simulink model "PositionComplementary"  (Simulink 6.6)
settings: Solver=ode4  StartTime=0.0  StopTime=60  FixedStep=SampleT  RelTol=1e-3
InitFcn:
  | clc
  | Taxi_Var_new
  | failures
  | insInit
  | piccolo_init
values from neighbouring files (symbols this model uses):
  A1 = 0    [Taxi_Var.m]    (also in Taxi_Var_new.m = 0.007)
  Apolar = 0.0899    [Taxi_Var.m]    (also in Taxi_Var_new.m = 0.057)
  CD0 = 0.0219    [Taxi_Var.m]    (also in Taxi_Var_new.m = 0.022)
  chord = S/span    (= 0.384036716878)    [Taxi_Var.m]    (also in Taxi_Var_new.m = 0.351341681574)
  CL0 = 0.1857    [Taxi_Var.m]    (also in Taxi_Var_new.m = 0.38)
  CLa = 4.6206    [Taxi_Var.m]    (also in Taxi_Var_new.m = 18.5)
  CLa_dot = 1.93    [Taxi_Var.m]    (also in Taxi_Var_new.m = 2.64)
  Clb = -0.0043    [Taxi_Var.m]    (also in Taxi_Var_new.m = -0.06)
  ClDa = 0.1695    [Taxi_Var.m]    (also in Taxi_Var_new.m)
  CLDe = 0.4032    [Taxi_Var.m]    (also in Taxi_Var_new.m = 0.24)
  CLDf = 0.047    [Taxi_Var.m]    (also in Taxi_Var_new.m = 0.4)
  ClDr = 0.0003    [Taxi_Var.m]    (also in Taxi_Var_new.m = 0.055)
  Clp = -0.4425    [Taxi_Var.m]    (also in Taxi_Var_new.m = -0.88)
  CLq = 8.7465    [Taxi_Var.m]    (also in Taxi_Var_new.m = 7.4)
  Clr = 0.0675    [Taxi_Var.m]    (also in Taxi_Var_new.m = 0.04)
  Cm0 = -0.0902    [Taxi_Var.m]    (also in Taxi_Var_new.m = 0.56)
  Cma = -1.3995    [Taxi_Var.m]    (also in Taxi_Var_new.m = -1.58)
  CmDe = -0.9493    [Taxi_Var.m]    (also in Taxi_Var_new.m = -41)
  CmDf = -.021    (= -0.021)    [Taxi_Var.m]    (also in Taxi_Var_new.m)
  Cmq = -10.8760    (= -10.876)    [Taxi_Var.m]    (also in Taxi_Var_new.m = -12)
  Cnb = 0.0281    [Taxi_Var.m]    (also in Taxi_Var_new.m = 0.73)
  CnDa = -0.0031    [Taxi_Var.m]    (also in Taxi_Var_new.m = -0.032)
  CnDr = -0.0882    [Taxi_Var.m]    (also in Taxi_Var_new.m = 0.19)
  Cnp = -0.0695    [Taxi_Var.m]    (also in Taxi_Var_new.m = -0.1)
  Cnr = -0.1045    [Taxi_Var.m]    (also in Taxi_Var_new.m = -0.23)
  CYb = -0.1999    [Taxi_Var.m]    (also in Taxi_Var_new.m = -0.98)
  CYDr = 0.0192    [Taxi_Var.m]    (also in Taxi_Var_new.m = 0.066)
  damax = 25*deg2rad    (= 0.436332312999)    [Taxi_Var.m]    (also in piccolo_init.m)
  damin = -25*deg2rad    (= -0.436332312999)    [Taxi_Var.m]    (also in piccolo_init.m)
  datrim = 0*deg2rad    (= 0)    [Taxi_Var.m]    (also in piccolo_init.m)
  demax = 15*deg2rad    (= 0.261799387799)    [Taxi_Var.m]    (also in piccolo_init.m)
  demin = -15*deg2rad    (= -0.261799387799)    [Taxi_Var.m]    (also in piccolo_init.m)
  detrim = -2.4137*deg2rad    (= -0.0421270121554)    [Taxi_Var.m]    (also in piccolo_init.m = -0.0523598775598)
  dfland = 30*deg2rad    (= 0.523598775598)    [Taxi_Var.m]    (also in piccolo_init.m)
  dfmax = 30*deg2rad    (= 0.523598775598)    [Taxi_Var.m]    (also in piccolo_init.m)
  dfmin = 0*deg2rad    (= 0)    [Taxi_Var.m]    (also in piccolo_init.m)
  drmax = 25*deg2rad    (= 0.436332312999)    [Taxi_Var.m]    (also in piccolo_init.m)
  drmin = -25*deg2rad    (= -0.436332312999)    [Taxi_Var.m]    (also in piccolo_init.m)
  drtrim = 0*deg2rad    (= 0)    [Taxi_Var.m]    (also in piccolo_init.m)
  dtmax = 1    [Taxi_Var.m]    (also in piccolo_init.m = 0.7)
  dtmin = 0    [Taxi_Var.m]    (also in piccolo_init.m = 0.25)
  dttrim = 0.0725    [Taxi_Var.m]    (also in piccolo_init.m = 0.35)
  Euler_0 = [0; 0; 45]'*pi/180    [Taxi_Var.m]    (also in Taxi_Var_new.m = [0 0 45]'*pi/180)
  IdxCmdOrbitRadius = 17    [piccolo_init.m]
  IdxCmdOrbitSense = 18    [piccolo_init.m]
  IdxCmdWp1Alt = 13    [piccolo_init.m]
  IdxCmdWp1Lat = 11    [piccolo_init.m]
  IdxCmdWp1Lon = 12    [piccolo_init.m]
  IdxCmdWp2Alt = 16    [piccolo_init.m]
  IdxCmdWp2Lat = 14    [piccolo_init.m]
  IdxCmdWp2Lon = 15    [piccolo_init.m]
  IdxEstimReserved1 = 4    [piccolo_init.m]
  IdxEstimWEast = 3    [piccolo_init.m]
  IdxEstimWNorth = 2    [piccolo_init.m]
  IdxGainsAltD = 10    [piccolo_init.m]
  IdxGainsAltI = 9    [piccolo_init.m]
  IdxGainsAltP = 8    [piccolo_init.m]
  IdxGainsPdynD = 4    [piccolo_init.m]
  IdxGainsPdynI = 3    [piccolo_init.m]
  IdxGainsPdynP = 2    [piccolo_init.m]
  IdxGainsPitchD = 7    [piccolo_init.m]
  IdxGainsPitchI = 6    [piccolo_init.m]
  IdxGainsPitchP = 5    [piccolo_init.m]
  IdxGainsRollD = 17    [piccolo_init.m]
  IdxGainsRollI = 16    [piccolo_init.m]
  IdxGainsRollP = 15    [piccolo_init.m]
  IdxGainsSlopeElevatorD = 25    [piccolo_init.m]
  IdxGainsSlopeElevatorP = 26    [piccolo_init.m]
  IdxGainsTrackConv = 24    [piccolo_init.m]
  IdxGainsTrackD = 23    [piccolo_init.m]
  IdxGainsTrackI = 22    [piccolo_init.m]
  IdxGainsTrackP = 21    [piccolo_init.m]
  IdxGainsTurnD = 14    [piccolo_init.m]
  IdxGainsTurnI = 13    [piccolo_init.m]
  IdxGainsTurnP = 12    [piccolo_init.m]
  IdxGainsYawD = 20    [piccolo_init.m]
  IdxGainsYawI = 19    [piccolo_init.m]
  IdxGainsYawP = 18    [piccolo_init.m]
  IdxLimitsAileronMax = 11    [piccolo_init.m]
  IdxLimitsAileronMin = 10    [piccolo_init.m]
  IdxLimitsBankMax = 9    [piccolo_init.m]
  IdxLimitsBankMin = 8    [piccolo_init.m]
  IdxLimitsElevatorMax = 13    [piccolo_init.m]
  IdxLimitsElevatorMin = 12    [piccolo_init.m]
  IdxLimitsFlapMax = 19    [piccolo_init.m]
  IdxLimitsFlapMin = 18    [piccolo_init.m]
  IdxLimitsPdynMax = 3    [piccolo_init.m]
  IdxLimitsPdynMin = 2    [piccolo_init.m]
  IdxLimitsRudderMax = 15    [piccolo_init.m]
  IdxLimitsRudderMin = 14    [piccolo_init.m]
  IdxLimitsThrottleMax = 17    [piccolo_init.m]
  IdxLimitsThrottleMin = 16    [piccolo_init.m]
  IdxSensorsAlt = 5    [piccolo_init.m]
  IdxSensorsLat = 3    [piccolo_init.m]
  IdxSensorsLon = 4    [piccolo_init.m]
  IdxSensorsVDown = 8    [piccolo_init.m]
  IdxSensorsVEast = 7    [piccolo_init.m]
  IdxSensorsVNorth = 6    [piccolo_init.m]
  IdxStatesGlobal = 2    [piccolo_init.m]
  IdxStatesManual = 16    [piccolo_init.m]
  IdxStatesMode = 15    [piccolo_init.m]
  ISA_g = 9.815    [Taxi_Var.m]    (also in Taxi_Var_new.m)
  ISA_hmax = 2000    [Taxi_Var.m]    (also in Taxi_Var_new.m)
  ISA_lapse = .0065    (= 0.0065)    [Taxi_Var.m]    (also in Taxi_Var_new.m)
  ISA_P0 = 101325    [Taxi_Var.m]    (also in Taxi_Var_new.m)
  ISA_R = 287    [Taxi_Var.m]    (also in Taxi_Var_new.m)
  ISA_rho0 = 1.225    [Taxi_Var.m]    (also in Taxi_Var_new.m)
  ISA_T0 = 289    [Taxi_Var.m]    (also in Taxi_Var_new.m)
  Ixx = 3.689084    [Taxi_Var.m]    (also in Taxi_Var_new.m = 3.8)
  Iyy = 7.43789    [Taxi_Var.m]    (also in Taxi_Var_new.m = 9.58)
  Izz = 10.22202    [Taxi_Var.m]    (also in Taxi_Var_new.m = 9.68)
  mass = 22.5    [Taxi_Var.m]    (also in Taxi_Var_new.m = 8.16466266)
  MinThK = 0.075    [Taxi_Var.m]    (also in Taxi_Var_new.m = 0.077)
  Pos_0 = [0; 0; 1000]'    [Taxi_Var.m]    (also in Taxi_Var_new.m = [0 0 500]')
  PQR_0 = [0; 0; 0]'    [Taxi_Var.m]    (also in Taxi_Var_new.m = [ 0 0 0]'*pi/180)
  SampleT = 0.005    [failures.m]
  span = 2.3368    [Taxi_Var.m]    (also in Taxi_Var_new.m = 2.795)
  TFact = 0.4    [Taxi_Var.m]    (also in Taxi_Var_new.m)
  ThK = 2.18    [Taxi_Var.m]    (also in Taxi_Var_new.m = 2.17)
  tsamp = APtsamp    (= 0.05)    [piccolo_init.m]
  ... (+1 more)
undefined symbols (not defined in the file or in its folder): clock, Earth, gaind, polesd, WGS84, zerosd
libraries: piccolo_library x60, simulink x45, aerolibconvert2 x13, dspsigops x5, aerolibasang x5, aerolibatmos2 x2, aerolibtransform2 x2, aerolibnav x2, aerolibutil x1, dspmtrx3 x1
(part 4 of 5)

== system PositionComplementary/Plant Model/Plant/6-DOF EOM/[V1,2,3,W1,2,3] ==
  note: V*dot =Inv(A){[F ; M] - SigmaAV*}
  "[F ; M]" : Inport
  Euler : Inport  Port=2
  V* : Inport  Port=3  PortDimensions=6
  A = [M ; J] : Subsystem
  Acc_meas : Product  Inputs=/*  Multiplication=Matrix(*)  SaturateOnIntegerOverflow=on  InputSameDT=on
  Demux : Demux  Outputs=[3;3]
  Get Grav Force in Body : Subsystem
  Gravitational Acc : Constant  Value=[0 0 -ISA_g]  VectorParams1D=off
  Reshape1 : Reshape
  Reshape2 : Reshape
  Scope : Scope
      settings: YMin=-90  YMax=10  SaveName=ScopeData34
  Selector3 : Selector  IndexOptions=Index vector (dialog)  Indices=1:3  OutputSizes=1  InputPortWidth=6
  Sigma : Subsystem
  Sigma*A : Product  Multiplication=Matrix(*)  SaturateOnIntegerOverflow=on  InputSameDT=on
  Sigma*A*V* : Product  Multiplication=Matrix(*)  SaturateOnIntegerOverflow=on  InputSameDT=on
  Sum1 : Sum  Inputs=+-|  SaturateOnIntegerOverflow=on  InputSameDT=on
  Sum2 : Sum  Inputs=++|  SaturateOnIntegerOverflow=on  InputSameDT=on
  Terminator1 : Terminator
  "V*dot " : Product  Inputs=/*  Multiplication=Matrix(*)  SaturateOnIntegerOverflow=on  InputSameDT=on
  "Acc_meas " : Outport
  V*dot : Outport  Port=2
  wires:
  Sum2/1 -> Reshape2/1
  Get Grav Force in Body/1(Grav Force (Body)) -> Reshape1/1
  Selector3/1 -> Sum2/2
  Euler/1 -> Get Grav Force in Body/1(Euler)
  Gravitational Acc/1 -> Get Grav Force in Body/2(Grav Force)
  Acc_meas/1 -> Selector3/1
  Sigma*A/1 -> Sigma*A*V*/1
  "V*dot "/1 -> V*dot/1
  V*/1 -> Demux/1, Sigma*A*V*/2
  Demux/2 -> Sigma/1(pqr)
  Sigma*A*V*/1 -> Sum1/2
  "[F ; M]"/1 -> Acc_meas/2, Sum1/1
  Sigma/1(Sigma) -> Sigma*A/1
  Demux/1 -> Terminator1/1
  A = [M ; J]/1(A Matrix) -> Acc_meas/1, "V*dot "/1, Sigma*A/2
  Sum1/1 -> "V*dot "/2
  Reshape1/1 -> Sum2/1
  Reshape2/1 -> "Acc_meas "/1, Scope/1

== system PositionComplementary/Plant Model/Plant/Engine Model/Get To1 ==
  dt : Inport
  Divide : Product  Inputs=3  OutScaling=2^-10
  Math Function : Math  Operator=pow  SaturateOnIntegerOverflow=on
  Math Function1 : Math  Operator=pow  SaturateOnIntegerOverflow=on
  MaxRPM : Gain  Gain=7200  SaturateOnIntegerOverflow=on
  Min RPM : Constant  Value=2000
  Min Th K : Constant  Value=MinThK
  Prop Diameter (in) : Constant  Value=17
  Prop Diameter (in)1 : Constant  Value=2
  Prop Diameter (in)2 : Constant  Value=4
  Saturation : Saturate  UpperLimit=1.0  LowerLimit=0.2
  Sum : Sum  Inputs=|++
  Sum1 : Sum  Inputs=|++
  TFact : simulink/Math Operations/Slider Gain  SystemSampleTime=-1  low=0  gain=0.2  high=1
  "TFact " : Gain  Gain=TFact  SaturateOnIntegerOverflow=on
  Th K : Gain  Gain=ThK  SaturateOnIntegerOverflow=on
  To Constant : Constant  Value=2.83e-12
  RPM : Outport
  To : Outport  Port=2
  wires:
  Saturation/1 -> Th K/1
  Prop Diameter (in)1/1 -> Math Function/2
  Prop Diameter (in)2/1 -> Math Function1/2
  Prop Diameter (in)/1 -> Math Function1/1
  Math Function/1 -> Divide/1
  Math Function1/1 -> Divide/2
  To Constant/1 -> Divide/3
  Divide/1 -> TFact/1
  TFact/1 -> To/1
  Sum/1 -> Math Function/1, RPM/1
  Min RPM/1 -> Sum/2
  MaxRPM/1 -> Sum/1
  Th K/1 -> Sum1/1
  dt/1 -> Saturation/1
  Sum1/1 -> MaxRPM/1
  Min Th K/1 -> Sum1/2

== system PositionComplementary/Plant Model/Plant/Forces and Moments/Alpha/Beta ==
  "Vx, Vy, Vz (Body)" : Inport
  Rho : Inport  Port=2
  Constant : Constant  Value=0.5  VectorParams1D=off
  Math Function : Math  Operator=sqrt  SaturateOnIntegerOverflow=on
  Product : Product  Inputs=3  SaturateOnIntegerOverflow=on
  Product1 : Product  Inputs=3  SaturateOnIntegerOverflow=on
  R2D1 : Gain  Gain=180/pi  SaturateOnIntegerOverflow=on
  R2D2 : Gain  Gain=180/pi  SaturateOnIntegerOverflow=on
  V^2 : Fcn  Expr=(u(1)^2+u(2)^2+u(3)^2)
  "[-15; 15 ]" : Saturate  UpperLimit=15  LowerLimit=-15
  "[-15;15]" : Saturate  UpperLimit=15  LowerLimit=-15
  aoa : Trigonometry  Operator=asin
  beta : Trigonometry  Operator=atan
  sin(aoa) : Fcn  Expr=u(3)/sqrt(u(1)^2+u(3)^2)
  span : Constant  Value=span  VectorParams1D=off
  span1 : Constant  Value=chord  VectorParams1D=off
  tan(beta) : Fcn  Expr=u(2)/sqrt(u(1)^2+u(3)^2)
  "alpha, deg" : Outport
  "beta, deg" : Outport  Port=2
  qS : Outport  Port=3
  Speed : Outport  Port=4
  q : Outport  Port=5
  wires:
  Product/1 -> q/1, Product1/1
  Product1/1 -> qS/1
  span1/1 -> Product1/3
  span/1 -> Product1/2
  "Vx, Vy, Vz (Body)"/1 -> sin(aoa)/1, V^2/1, tan(beta)/1
  tan(beta)/1 -> beta/1
  beta/1 -> R2D1/1
  V^2/1 -> Product/1, Math Function/1
  Rho/1 -> Product/2
  Constant/1 -> Product/3
  R2D1/1 -> "[-15; 15 ]"/1  "beta"
  aoa/1 -> R2D2/1
  R2D2/1 -> "[-15;15]"/1  "aoa"
  sin(aoa)/1 -> aoa/1
  Math Function/1 -> Speed/1
  "[-15;15]"/1 -> "alpha, deg"/1
  "[-15; 15 ]"/1 -> "beta, deg"/1

== system PositionComplementary/Plant Model/Plant/Forces and Moments/Body Frame F & M ==
  "Alpha, deg" : Inport
  "Beta, deg" : Inport  Port=2
  qs : Inport  Port=3
  Airspeed : Inport  Port=4
  "de, deg" : Inport  Port=5
  "da, deg" : Inport  Port=6
  "dr, deg" : Inport  Port=7
  "df, deg" : Inport  Port=8
  p,q,r : Inport  Port=9
  Bus Creator : BusCreator  Inputs=2
  Transfer to body frame : Subsystem
  Wind frame F& M : Subsystem
  F_b : Outport
  M_b : Outport  Port=2
  wires:
  "Alpha, deg"/1 -> Wind frame F& M/1("alpha, deg"), Bus Creator/1
  "Beta, deg"/1 -> Wind frame F& M/2("beta, deg"), Bus Creator/2
  "dr, deg"/1 -> Wind frame F& M/5("dr, deg")
  "da, deg"/1 -> Wind frame F& M/4("da, deg")
  "de, deg"/1 -> Wind frame F& M/3("de, deg")
  Wind frame F& M/1(F&M wind frame) -> Transfer to body frame/1(Wind frame  F&M)
  Bus Creator/1 -> Transfer to body frame/2("aoa/beta, deg")  "aoa/beta, deg"
  Transfer to body frame/1(F_b) -> F_b/1
  Transfer to body frame/2(M_b) -> M_b/1
  "df, deg"/1 -> Wind frame F& M/6("df, deg")
  qs/1 -> Wind frame F& M/7(qS)
  p,q,r/1 -> Wind frame F& M/8(p,q,r)
  Airspeed/1 -> Wind frame F& M/9(Airpseed)

== system PositionComplementary/Plant Model/Plant/Forces and Moments/Get Grav Force in Body ==
  Euler : Inport
  Grav Force : Inport  Port=2
  Math Function : Math  Operator=transpose  SaturateOnIntegerOverflow=on
  Product1 : Product  Multiplication=Matrix(*)  SaturateOnIntegerOverflow=on  InputSameDT=on
  Rb2u : Subsystem
  Reshape : Reshape  OutputDimensionality=Column vector (2-D)
  Grav Force (Body) : Outport
  wires:
  Rb2u/1(DCM) -> Math Function/1
  Euler/1 -> Rb2u/1(phi theta psi)
  Product1/1 -> Grav Force (Body)/1
  Math Function/1 -> Product1/1
  Grav Force/1 -> Reshape/1
  Reshape/1 -> Product1/2

== system PositionComplementary/Plant Model/Plant/Forces and Moments/NED(u)2b ==
  V w : Inport
  Euler : Inport  Port=2
  RB2LTP : Subsystem
  RL2B * Vw : Product  Multiplication=Matrix(*)  SaturateOnIntegerOverflow=on  InputSameDT=on
  RLTP2B : Math  Operator=transpose  SaturateOnIntegerOverflow=on
  Reshape1 : Reshape  OutputDimensionality=Row vector (2-D)
  Vb Corr : Outport
  wires:
  RL2B * Vw/1 -> Reshape1/1
  Euler/1 -> RB2LTP/1(Euler)
  RB2LTP/1(RB2L) -> RLTP2B/1
  RLTP2B/1 -> RL2B * Vw/1
  V w/1 -> RL2B * Vw/2
  Reshape1/1 -> Vb Corr/1

== system PositionComplementary/Signal Cond/Accel Convert/3vector LPF/Low Pass1 ==
  In1 : Inport
  Discrete Zero-Pole : DiscreteZeroPole  Zeros=zerosd  Poles=polesd  Gain=gaind  SampleTime=SampleTime
  Out1 : Outport
  wires:
  In1/1 -> Discrete Zero-Pole/1
  Discrete Zero-Pole/1 -> Out1/1

== system PositionComplementary/Signal Cond/Accel Convert/3vector LPF/Low Pass2 ==
  In1 : Inport
  Discrete Zero-Pole : DiscreteZeroPole  Zeros=zerosd  Poles=polesd  Gain=gaind  SampleTime=SampleTime
  Out1 : Outport
  wires:
  Discrete Zero-Pole/1 -> Out1/1
  In1/1 -> Discrete Zero-Pole/1

== system PositionComplementary/Signal Cond/Accel Convert/3vector LPF/Low Pass3 ==
  In1 : Inport
  Discrete Zero-Pole : DiscreteZeroPole  Zeros=zerosd  Poles=polesd  Gain=gaind  SampleTime=SampleTime
  Out1 : Outport
  wires:
  In1/1 -> Discrete Zero-Pole/1
  Discrete Zero-Pole/1 -> Out1/1

== system PositionComplementary/Signal Cond/Gyro Convert/3vector LPF/Low Pass1 ==
  In1 : Inport
  Discrete Zero-Pole : DiscreteZeroPole  Zeros=zerosd  Poles=polesd  Gain=gaind  SampleTime=SampleTime
  Out1 : Outport
  wires:
  In1/1 -> Discrete Zero-Pole/1
  Discrete Zero-Pole/1 -> Out1/1

== system PositionComplementary/Signal Cond/Gyro Convert/3vector LPF/Low Pass2 ==
  In1 : Inport
  Discrete Zero-Pole : DiscreteZeroPole  Zeros=zerosd  Poles=polesd  Gain=gaind  SampleTime=SampleTime
  Out1 : Outport
  wires:
  Discrete Zero-Pole/1 -> Out1/1
  In1/1 -> Discrete Zero-Pole/1

== system PositionComplementary/Signal Cond/Gyro Convert/3vector LPF/Low Pass3 ==
  In1 : Inport
  Discrete Zero-Pole : DiscreteZeroPole  Zeros=zerosd  Poles=polesd  Gain=gaind  SampleTime=SampleTime
  Out1 : Outport
  wires:
  In1/1 -> Discrete Zero-Pole/1
  Discrete Zero-Pole/1 -> Out1/1

== system PositionComplementary/Subsystem3/Autopilot/Altitude Control Vector Inputs/Alt switch ==
  note: Select whether the individual components of the altitude, airspeed and turn rate loops are enabled or
      | disabled.  This is done based on the specific loop enable state, the global state, and the mode of the autopilot.
      |
      | Note the use of the multiport  switch.  This switch is one based, and will truncate floating point
      | numbers.  Hence we add by 1.1 to guarantee we don't get the wrong state based on rounding
      | error.
  Globals : Inport
  Loop : Inport  Port=2
  Climbout : Constant
  Convert to 1 based : Constant  Value=1.1
  Default : Constant
  Demux : Demux  Outputs=3
  Display4 : Display
  Final Approach : Constant
  Flying : Constant
  Global and Loop on/off : Product  SaturateOnIntegerOverflow=on
  Land pattern : Constant
  Loop on or off : Switch  Threshold=0.5  SaturateOnIntegerOverflow=on
  Mux : Mux  Inputs=3
  Mux1 : Mux  Inputs=3
  PID switch : MultiPortSwitch  Inputs=8  SaturateOnIntegerOverflow=on  InputSameDT=on
  Pre launch : Constant  Value=0
  Sum : Sum  Inputs=++|  SaturateOnIntegerOverflow=on  InputSameDT=on
  Terminator : Terminator
  Touchdown : Constant
  Transition : Constant  Value=0
  Zero : Constant  Value=0
  TriOut : Outport  OutDataType=fixdt(1,16,0)  OutScaling=[]
  wires:
  Sum/1 -> PID switch/1
  Default/1 -> PID switch/9
  Touchdown/1 -> PID switch/8
  Final Approach/1 -> PID switch/7
  Land pattern/1 -> PID switch/6
  Flying/1 -> PID switch/5
  Transition/1 -> PID switch/3
  Climbout/1 -> PID switch/4
  Pre launch/1 -> PID switch/2
  Demux/3 -> Terminator/1
  Mux1/1 -> Loop on or off/1
  PID switch/1 -> Mux1/3, Mux1/2, Mux1/1
  Convert to 1 based/1 -> Sum/1
  Demux/2 -> Sum/2
  Global and Loop on/off/1 -> Loop on or off/2
  Loop/1 -> Global and Loop on/off/2
  Demux/1 -> Global and Loop on/off/1
  Globals/1 -> Demux/1, Display4/1
  Zero/1 -> Mux/3, Mux/2, Mux/1
  Mux/1 -> Loop on or off/3
  Loop on or off/1 -> TriOut/1

== system PositionComplementary/Subsystem3/Autopilot/Altitude Control Vector Inputs/Integral Gain  Scheduling ==
  note: 3. Then the IntegralGain2 = IntegralGain * GainScheduleFactor
  note: 2. We compute GainScheduleFactor = exp(-error^2 / (2*sigma^2))
  note: 1. We compute sigma = ScalingParam * ActuatorRange/2 / Kp
  note: Integral gain scheduling based on a Gaussian distribution, as a function of the error, actuator range, and proportional gain.
  err : Inport
  Gains : Inport  Port=2
  Limits : Inport  Port=3
  Demux : Demux  Outputs=2
  Demux1 : Demux  Outputs=3
  Gain : Gain  Gain=0.5  SaturateOnIntegerOverflow=on
  Gain1 : Gain  Gain=2  SaturateOnIntegerOverflow=on
  Gain2 : Gain  Gain=-1  SaturateOnIntegerOverflow=on
  Math Function : Math  Operator=square  OutDataType=fixdt(1,16,0)  OutScaling=[]  SaturateOnIntegerOverflow=on
  Math Function1 : Math  Operator=square  OutDataType=fixdt(1,16,0)  OutScaling=[]  SaturateOnIntegerOverflow=on
  Math Function2 : Math  OutDataType=fixdt(1,16,0)  OutScaling=[]  SaturateOnIntegerOverflow=on
  Mux1 : Mux  Inputs=3
  Product : Product  Inputs=/**  SaturateOnIntegerOverflow=on
  Product1 : Product  Inputs=*/  SaturateOnIntegerOverflow=on
  Product2 : Product  SaturateOnIntegerOverflow=on
  Scaling param : Constant  Value=0.5
  Sum : Sum  Inputs=+-  SaturateOnIntegerOverflow=on
  Zero Protect : piccolo_library/Math/Zero Protect  SystemSampleTime=-1  p=1  tol=1e-6
  Gains2 : Outport  OutDataType=fixdt(1,16,0)  OutScaling=[]
  wires:
  Zero Protect/1 -> Product/1
  Demux1/1 -> Mux1/1, Zero Protect/1
  Demux1/3 -> Mux1/3
  Product2/1 -> Mux1/2
  Mux1/1 -> Gains2/1
  Demux1/2 -> Product2/2
  Gains/1 -> Demux1/1
  Math Function2/1 -> Product2/1
  Product1/1 -> Math Function2/1
  Gain1/1 -> Product1/2
  Gain2/1 -> Product1/1
  Math Function1/1 -> Gain2/1
  err/1 -> Math Function1/1
  Math Function/1 -> Gain1/1
  Product/1 -> Math Function/1
  Scaling param/1 -> Product/3
  Gain/1 -> Product/2
  Sum/1 -> Gain/1
  Demux/2 -> Sum/2
  Demux/1 -> Sum/1
  Limits/1 -> Demux/1

== system PositionComplementary/Subsystem3/Autopilot/Altitude Control Vector Inputs/Min alt ==
  note: Determin the min altitude to use. Either -10000 or the passed in value, depending on if Auto land is enabled
  Globals : Inport
  MinAlt : Inport  Port=2
  -10000 : Constant  Value=-10000
  Climbout : Constant  Value=0
  Convert to 1 based : Constant  Value=1.1
  Default : Constant  Value=0
  Demux : Demux  Outputs=3
  Final Approach : Constant
  Flying : Constant  Value=0
  Land pattern : Constant
  Loop on or off : Switch  Threshold=0.5  SaturateOnIntegerOverflow=on
  Min alt on/off : MultiPortSwitch  Inputs=8  SaturateOnIntegerOverflow=on  InputSameDT=on
  Pre launch : Constant  Value=0
  Sum : Sum  Inputs=++|  SaturateOnIntegerOverflow=on  InputSameDT=on
  Terminator : Terminator
  Terminator1 : Terminator
  Touchdown : Constant
  Transition : Constant  Value=0
  MinAltOut : Outport  OutDataType=fixdt(1,16,0)  OutScaling=[]
  wires:
  Sum/1 -> Min alt on/off/1
  Default/1 -> Min alt on/off/9
  Touchdown/1 -> Min alt on/off/8
  Final Approach/1 -> Min alt on/off/7
  Land pattern/1 -> Min alt on/off/6
  Flying/1 -> Min alt on/off/5
  Transition/1 -> Min alt on/off/3
  Climbout/1 -> Min alt on/off/4
  Pre launch/1 -> Min alt on/off/2
  -10000/1 -> Loop on or off/1
  Min alt on/off/1 -> Loop on or off/2
  Loop on or off/1 -> MinAltOut/1
  Globals/1 -> Demux/1
  Demux/1 -> Terminator1/1
  MinAlt/1 -> Loop on or off/3
  Demux/2 -> Sum/2
  Convert to 1 based/1 -> Sum/1
  Demux/3 -> Terminator/1

== system PositionComplementary/Subsystem3/Autopilot/Altitude Control Vector Inputs/PID Controller ==
  note: Standard PID feedback controller with integrator saturation. There are three gains, and three states, one for each term
  Input : Inport
  Cmd : Inport  Port=2
  State : Inport  Port=3
  Gains : Inport  Port=4
  Limits : Inport  Port=5
  IniCond : Inport  Port=6
  Demux : Demux  Outputs=3
  Demux1 : Demux  Outputs=3
  Derivative Gain : Product  Inputs=3  SaturateOnIntegerOverflow=on  InputSameDT=on
  Extended Integrator : Subsystem  AncestorBlock=piccolo_library/Integrators/Extended Integrator  mask(Extended Integrator){T=tsamp}
      mask prompts: T "Sample time:"
      mask help:
      | Trapezoidal integration with integrator reset and anti-windup logic
      | The block computes the integral.  The integrator gets the IC value
      | whenever the enable line is down.  Anytime the enable line is
      | down the output is the IC value.  If the gain goes to zero then the
      | integrator value is reset.
  Proportional Gain : Product  Inputs=3  SaturateOnIntegerOverflow=on  InputSameDT=on
  Scope1 : Scope  NumInputPorts=3
      settings: YMin=0.045~0.038~-1  YMax=0.051~0.058~1  SaveName=ScopeData32
  Scope2 : Scope  NumInputPorts=3
      settings: YMin=0.045~0.038~-1  YMax=0.051~0.058~1  SaveName=ScopeData20
  Sum : Sum  Inputs=|+-  SaturateOnIntegerOverflow=on
  Sum3 : Sum  Inputs=+++  SaturateOnIntegerOverflow=on  InputSameDT=on
  dx/dt with TD : piccolo_library/Derivatives/dx//dt with TD  SystemSampleTime=-1  tsamp=tsamp  tdelay=tdelay
  Output : Outport  OutDataType=fixdt(1,16,0)  OutScaling=[]
  wires:
  Sum3/1 -> Output/1
  Demux1/3 -> Derivative Gain/3
  Demux1/2 -> Extended Integrator/3(Enable)
  Demux1/1 -> Proportional Gain/3
  State/1 -> Demux1/1
  IniCond/1 -> Extended Integrator/2(IniCond)
  Limits/1 -> Extended Integrator/5(Limits)
  Demux/2 -> Extended Integrator/4(Gain)
  Extended Integrator/1(Out) -> Sum3/2, Scope2/2
  Derivative Gain/1 -> Sum3/3, Scope2/3
  Proportional Gain/1 -> Sum3/1, Scope2/1
  Demux/3 -> Derivative Gain/2
  Demux/1 -> Proportional Gain/2
  Gains/1 -> Demux/1
  dx/dt with TD/1 -> Derivative Gain/1
  Sum/1 -> Extended Integrator/1(Input), dx/dt with TD/1, Proportional Gain/1
  Cmd/1 -> Sum/2, Scope1/1, Scope1/2
  Input/1 -> Sum/1

== system PositionComplementary/Subsystem3/Autopilot/Altitude Control Vector Inputs/Total Energy1 ==
  TAS : Inport
  Alt : Inport  Port=2
  TASCmd : Inport  Port=3
  AltCmd : Inport  Port=4
  State : Inport  Port=5
  1/2 : Constant  Value=0.5
  Kinetic : Product  Inputs=***  SaturateOnIntegerOverflow=on  InputSameDT=on
  Kinetic1 : Product  Inputs=*/  SaturateOnIntegerOverflow=on  InputSameDT=on
  Kinetic2 : Product  Inputs=***  SaturateOnIntegerOverflow=on  InputSameDT=on
  Sum1 : Sum  SaturateOnIntegerOverflow=on  InputSameDT=on
  Sum2 : Sum  SaturateOnIntegerOverflow=on  InputSameDT=on
  Switch : Switch  Threshold=0.5  SaturateOnIntegerOverflow=on
  Switch1 : Switch  Threshold=0.5  SaturateOnIntegerOverflow=on
  Zero : Constant  Value=0.0
  g1 : Constant  Value=9.806
  Energy : Outport  OutDataType=fixdt(1,16,0)  OutScaling=[]
  Cmd : Outport  Port=2  OutDataType=fixdt(1,16,0)  OutScaling=[]
  wires:
  TASCmd/1 -> Kinetic2/3, Kinetic2/2
  Sum1/1 -> Cmd/1
  AltCmd/1 -> Sum1/2
  Switch1/1 -> Sum1/1
  Kinetic2/1 -> Switch1/1
  Sum2/1 -> Energy/1
  Alt/1 -> Sum2/1
  Switch/1 -> Sum2/2
  Kinetic1/1 -> Kinetic2/1, Kinetic/3
  1/2/1 -> Kinetic1/1
  g1/1 -> Kinetic1/2
  Kinetic/1 -> Switch/1
  State/1 -> Switch/2, Switch1/2
  Zero/1 -> Switch/3, Switch1/3
  TAS/1 -> Kinetic/1, Kinetic/2

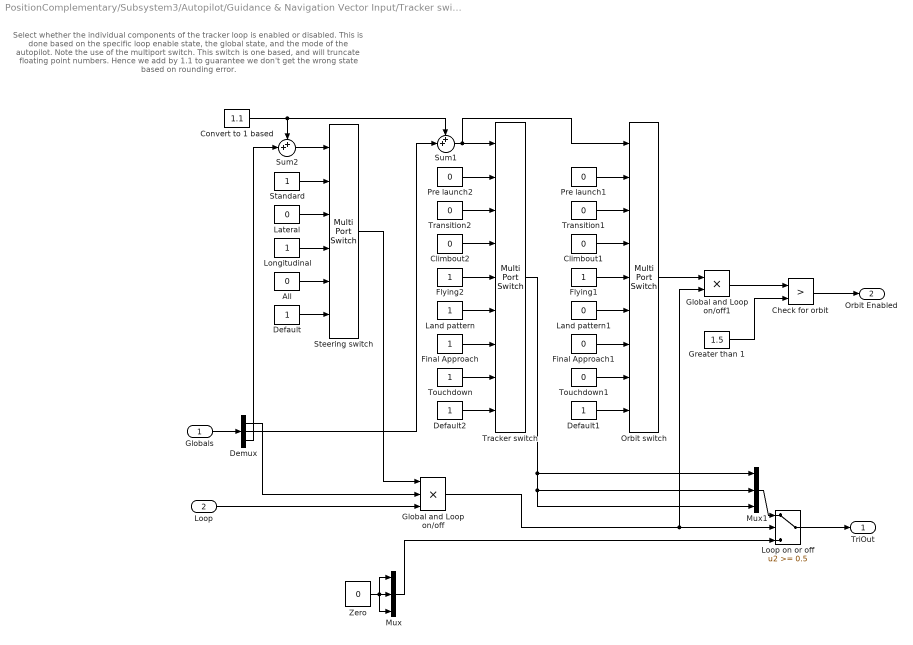
== system PositionComplementary/Subsystem3/Autopilot/Guidance & Navigation Vector Input/Tracker switch ==
  note: Select whether the individual components of the tracker loop is enabled or
      | disabled.  This is done based on the specific loop enable state, the global state, and the mode of the autopilot.
      |
      | Note the use of the multiport  switch.  This switch is one based, and will truncate floating point
      | numbers.  Hence we add by 1.1 to guarantee we don't get the wrong state based on rounding
      | error.
  Globals : Inport
  Loop : Inport  Port=2
  All : Constant  Value=0
  Check for orbit : RelationalOperator  Operator=>
  Climbout1 : Constant  Value=0
  Climbout2 : Constant  Value=0
  Convert to 1 based : Constant  Value=1.1
  Default : Constant
  Default1 : Constant
  Default2 : Constant
  Demux : Demux  Outputs=3
  Final Approach : Constant
  Final Approach1 : Constant  Value=0
  Flying1 : Constant
  Flying2 : Constant
  Global and Loop on/off : Product  Inputs=3  SaturateOnIntegerOverflow=on
  Global and Loop on/off1 : Product  SaturateOnIntegerOverflow=on
  Greater than 1 : Constant  Value=1.5
  Land pattern : Constant
  Land pattern1 : Constant  Value=0
  Lateral : Constant  Value=0
  Longitudinal : Constant
  Loop on or off : Switch  Threshold=0.5  SaturateOnIntegerOverflow=on
  Mux : Mux  Inputs=3
  Mux1 : Mux  Inputs=3
  Orbit switch : MultiPortSwitch  Inputs=8  SaturateOnIntegerOverflow=on  InputSameDT=on
  Pre launch1 : Constant  Value=0
  Pre launch2 : Constant  Value=0
  Standard : Constant
  Steering switch : MultiPortSwitch  Inputs=5  SaturateOnIntegerOverflow=on  InputSameDT=on
  Sum1 : Sum  Inputs=++|  SaturateOnIntegerOverflow=on  InputSameDT=on
  Sum2 : Sum  Inputs=++|  SaturateOnIntegerOverflow=on  InputSameDT=on
  Touchdown : Constant
  Touchdown1 : Constant  Value=0
  Tracker switch : MultiPortSwitch  Inputs=8  SaturateOnIntegerOverflow=on  InputSameDT=on
  Transition1 : Constant  Value=0
  Transition2 : Constant  Value=0
  Zero : Constant  Value=0
  TriOut : Outport  OutDataType=fixdt(1,16,0)  OutScaling=[]
  Orbit Enabled : Outport  Port=2  OutDataType=fixdt(1,16,0)  OutScaling=[]
  wires:
  Steering switch/1 -> Global and Loop on/off/1
  Demux/1 -> Global and Loop on/off/2
  Loop/1 -> Global and Loop on/off/3
  Sum2/1 -> Steering switch/1
  Default/1 -> Steering switch/6
  All/1 -> Steering switch/5
  Lateral/1 -> Steering switch/3
  Longitudinal/1 -> Steering switch/4
  Standard/1 -> Steering switch/2
  Convert to 1 based/1 -> Sum2/1, Sum1/1
  Default1/1 -> Orbit switch/9
  Touchdown1/1 -> Orbit switch/8
  Final Approach1/1 -> Orbit switch/7
  Land pattern1/1 -> Orbit switch/6
  Flying1/1 -> Orbit switch/5
  Transition1/1 -> Orbit switch/3
  Climbout1/1 -> Orbit switch/4
  Pre launch1/1 -> Orbit switch/2
  Sum1/1 -> Orbit switch/1, Tracker switch/1
  Default2/1 -> Tracker switch/9
  Touchdown/1 -> Tracker switch/8
  Final Approach/1 -> Tracker switch/7
  Land pattern/1 -> Tracker switch/6
  Flying2/1 -> Tracker switch/5
  Transition2/1 -> Tracker switch/3
  Climbout2/1 -> Tracker switch/4
  Pre launch2/1 -> Tracker switch/2
  Mux1/1 -> Loop on or off/1
  Tracker switch/1 -> Mux1/2, Mux1/3, Mux1/1
  Zero/1 -> Mux/3, Mux/2, Mux/1
  Mux/1 -> Loop on or off/3
  Check for orbit/1 -> Orbit Enabled/1
  Greater than 1/1 -> Check for orbit/2
  Orbit switch/1 -> Global and Loop on/off1/1
  Global and Loop on/off1/1 -> Check for orbit/1
  Demux/3 -> Sum2/2
  Demux/2 -> Sum1/2
  Global and Loop on/off/1 -> Global and Loop on/off1/2, Loop on or off/2
  Globals/1 -> Demux/1
  Loop on or off/1 -> TriOut/1

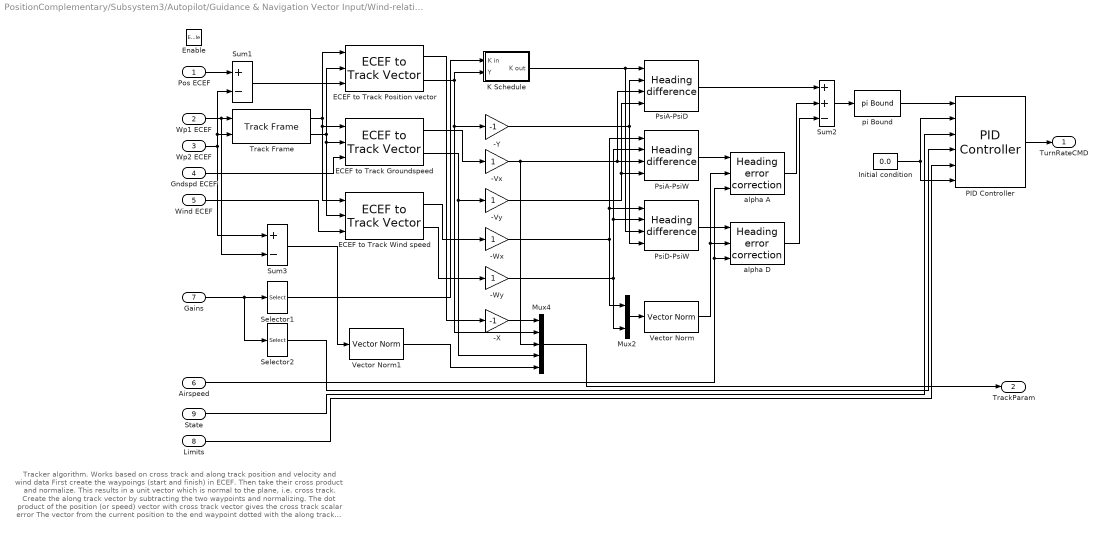
== system PositionComplementary/Subsystem3/Autopilot/Guidance & Navigation Vector Input/Wind-relative Tracker ==
  note: Tracker algorithm.  Works based on cross track and along track position and velocity and wind data
      |
      | First create the waypoings (start and finish) in ECEF.  Then take their cross product and normalize.  This results in a unit vector which is normal to the plane, i.e. cross track.
      | Create the along track vector by subtracting the two waypoints and normalizing.
      | The dot product of the position (or speed) vector with cross track vector gives the cross track scalar error
      | The vector from the current position to the end waypoint dotted with the along track vector gives the along track value
  Pos ECEF : Inport
  Wp1 ECEF : Inport  Port=2
  Wp2 ECEF : Inport  Port=3
  Gndspd ECEF : Inport  Port=4
  Wind ECEF : Inport  Port=5
  Airspeed : Inport  Port=6
  Gains : Inport  Port=7
  Limits : Inport  Port=8
  State : Inport  Port=9
  Enable : EnablePort
  -Vx : Gain  SaturateOnIntegerOverflow=on
  -Vy : Gain  SaturateOnIntegerOverflow=on
  -Wx : Gain  SaturateOnIntegerOverflow=on
  -Wy : Gain  SaturateOnIntegerOverflow=on
  -X : Gain  Gain=-1  SaturateOnIntegerOverflow=on
  -Y : Gain  Gain=-1  SaturateOnIntegerOverflow=on
  ECEF to Track Groundspeed : piccolo_library/Transformations/ECEF to Track Vector  SystemSampleTime=-1
  ECEF to Track Position vector : piccolo_library/Transformations/ECEF to Track Vector  SystemSampleTime=-1
  ECEF to Track Wind speed : piccolo_library/Transformations/ECEF to Track Vector  SystemSampleTime=-1
  Initial condition : Constant  Value=0.0
  K Schedule : Subsystem
  Mux2 : Mux  Inputs=2
  Mux4 : Mux  Inputs=5
  PID Controller : piccolo_library/Controllers/PID Controller  SystemSampleTime=-1  tsamp=tsamp  tdelay=tsamp
  PsiA-PsiD : piccolo_library/Controllers/Guidance/Heading difference  SystemSampleTime=-1
  PsiA-PsiW : piccolo_library/Controllers/Guidance/Heading difference  SystemSampleTime=-1
  PsiD-PsiW : piccolo_library/Controllers/Guidance/Heading difference  SystemSampleTime=-1
  Selector1 : Selector  IndexOptions=Index vector (dialog)  Indices=[4]  OutputSizes=1  InputPortWidth=4
  Selector2 : Selector  IndexOptions=Index vector (dialog)  Indices=[1 2 3]  OutputSizes=1  InputPortWidth=4
  Sum1 : Sum  Inputs=+-  SaturateOnIntegerOverflow=on  InputSameDT=on
  Sum2 : Sum  Inputs=++-  SaturateOnIntegerOverflow=on  InputSameDT=on
  Sum3 : Sum  Inputs=+-  SaturateOnIntegerOverflow=on  InputSameDT=on
  Track Frame : piccolo_library/Transformations/Track Frame  SystemSampleTime=-1
  Vector Norm : piccolo_library/Math/Vector Norm  SystemSampleTime=-1
  Vector Norm1 : piccolo_library/Math/Vector Norm  SystemSampleTime=-1
  alpha A : piccolo_library/Controllers/Guidance/Heading error correction  SystemSampleTime=-1
  alpha D : piccolo_library/Controllers/Guidance/Heading error correction  SystemSampleTime=-1
  pi Bound : piccolo_library/Math/pi Bound  SystemSampleTime=-1
  TurnRateCMD : Outport  OutDataType=fixdt(1,16,0)  OutScaling=[]
  TrackParam : Outport  Port=2  OutDataType=fixdt(1,16,0)  OutScaling=[]
  wires:
  Sum3/1 -> Vector Norm1/1
  Vector Norm1/1 -> Mux4/5
  -Y/1 -> PsiD-PsiW/4, PsiA-PsiD/2
  K Schedule/1(K out) -> PsiA-PsiD/1, PsiD-PsiW/3
  PID Controller/1 -> TurnRateCMD/1
  Initial condition/1 -> PID Controller/2, PID Controller/6
  -X/1 -> Mux4/1
  ECEF to Track Wind speed/1 -> -Wx/1
  ECEF to Track Wind speed/2 -> -Wy/1
  ECEF to Track Groundspeed/2 -> Mux4/4, -Vy/1
  ECEF to Track Groundspeed/1 -> -Vx/1
  ECEF to Track Position vector/1 -> -X/1
  ECEF to Track Position vector/2 -> -Y/1, Mux4/2, K Schedule/2(Y)
  Selector1/1 -> K Schedule/1(K in)
  Mux2/1 -> Vector Norm/1
  Vector Norm/1 -> alpha D/2, alpha A/2
  -Wy/1 -> Mux2/2, PsiD-PsiW/2, PsiA-PsiW/2
  -Vy/1 -> PsiA-PsiD/4, PsiA-PsiW/4
  -Wx/1 -> Mux2/1, PsiD-PsiW/1, PsiA-PsiW/1
  -Vx/1 -> Mux4/3, PsiA-PsiD/3, PsiA-PsiW/3
  pi Bound/1 -> PID Controller/1
  Sum2/1 -> pi Bound/1
  alpha D/1 -> Sum2/3
  alpha A/1 -> Sum2/2
  PsiA-PsiD/1 -> Sum2/1
  Limits/1 -> PID Controller/5
  State/1 -> PID Controller/3
  PsiD-PsiW/1 -> alpha D/1
  PsiA-PsiW/1 -> alpha A/1
  Mux4/1 -> TrackParam/1
  Selector2/1 -> PID Controller/4
  Airspeed/1 -> alpha D/3, alpha A/3
  Gains/1 -> Selector2/1, Selector1/1
  Wind ECEF/1 -> ECEF to Track Wind speed/3
  Gndspd ECEF/1 -> ECEF to Track Groundspeed/3
  Track Frame/2 -> ECEF to Track Wind speed/2, ECEF to Track Groundspeed/2, ECEF to Track Position vector/2
  Track Frame/1 -> ECEF to Track Wind speed/1, ECEF to Track Groundspeed/1, ECEF to Track Position vector/1
  Sum1/1 -> ECEF to Track Position vector/3
  Pos ECEF/1 -> Sum1/1
  Wp2 ECEF/1 -> Sum3/1, Sum1/2, Track Frame/2
  Wp1 ECEF/1 -> Sum3/2, Track Frame/1

== system PositionComplementary/Subsystem3/Autopilot/Pitch Control  Vector Inputs/PDynCmd ==
  AltError : Inport
  QCmd : Inport  Port=2
  QShift : Inport  Port=3
  QLimits : Inport  Port=4
  States : Inport  Port=5
  Density : Inport  Port=6
  -0.2 : Gain  Gain=-.2  SaturateOnIntegerOverflow=on
  0.3 : Gain  Gain=.3  SaturateOnIntegerOverflow=on
  1-based : Constant  Value=1.1
  All : Constant  Value=0
  Default : Constant  Value=0
  Enabled? : Logic  AllPortsSameDT=off
  Energy or not? : Switch  Threshold=0.5  SaturateOnIntegerOverflow=on
  Gravity : Gain  Gain=9.8  SaturateOnIntegerOverflow=on
  Lateral : Constant
  Limited QShift : piccolo_library/Nonlinear/SaturationEx  SystemSampleTime=-1
  Longitudinal : Constant  Value=0
  Manual assist switch : MultiPortSwitch  Inputs=5  SaturateOnIntegerOverflow=on  InputSameDT=on
  Mux : Mux  Inputs=2
  PDyn saturation : piccolo_library/Nonlinear/SaturationEx  SystemSampleTime=-1
  PDyn saturation1 : piccolo_library/Nonlinear/SaturationEx  SystemSampleTime=-1
  Qshift : Product  SaturateOnIntegerOverflow=on
  Selector1 : Selector  IndexOptions=Index vector (dialog)  Indices=IdxStatesManual  OutputSizes=1  InputPortWidth=SizeStates
  Selector2 : Selector  IndexOptions=Index vector (dialog)  Indices=IdxStatesAltToPdyn  OutputSizes=1  InputPortWidth=SizeStates
  Standard : Constant
  Sum : Sum  Inputs=|++  SaturateOnIntegerOverflow=on
  Sum1 : Sum  SaturateOnIntegerOverflow=on
  QCmdOut : Outport  OutDataType=fixdt(1,16,0)  OutScaling=[]
  QCmdNom : Outport  Port=2  OutDataType=fixdt(1,16,0)  OutScaling=[]
  wires:
  Enabled?/1 -> Energy or not?/2
  Manual assist switch/1 -> Enabled?/1
  Selector2/1 -> Enabled?/2
  PDyn saturation1/1 -> QCmdNom/1
  Sum1/1 -> PDyn saturation/1
  Energy or not?/1 -> Sum1/2
  QLimits/1 -> PDyn saturation1/2, PDyn saturation/2
  PDyn saturation/1 -> QCmdOut/1
  QShift/1 -> Energy or not?/3
  Limited QShift/1 -> Energy or not?/1
  Sum/1 -> Manual assist switch/1
  1-based/1 -> Sum/2
  Selector1/1 -> Sum/1
  States/1 -> Selector2/1, Selector1/1
  Default/1 -> Manual assist switch/6
  All/1 -> Manual assist switch/5
  Lateral/1 -> Manual assist switch/3
  Longitudinal/1 -> Manual assist switch/4
  Standard/1 -> Manual assist switch/2
  QCmd/1 -> PDyn saturation1/1, Sum1/1, -0.2/1, 0.3/1
  Qshift/1 -> Limited QShift/1
  Mux/1 -> Limited QShift/2
  0.3/1 -> Mux/2
  -0.2/1 -> Mux/1
  Gravity/1 -> Qshift/1
  AltError/1 -> Gravity/1
  Density/1 -> Qshift/2

== system PositionComplementary/Subsystem3/Autopilot/Pitch Control  Vector Inputs/Pdyn Hold ==
  Input : Inport
  Cmd : Inport  Port=2
  State : Inport  Port=3
  Gains : Inport  Port=4
  Limits : Inport  Port=5
  Actuator Trim : Inport  Port=6
  50 [Pa/s] : Constant  Value=100
  PID Controller : Subsystem  AncestorBlock=piccolo_library/Controllers/PID Controller  mask(PID Controller){tsamp=tsamp, tdelay=0.5}
      mask prompts: tsamp "Sample time:"; tdelay "Time derivative delay:"
      mask help: Generic PID (proportional, integral, derivative) controller with a single input and a single output.
  Rate Limit Ex : piccolo_library/Nonlinear/Rate Limit Ex  SystemSampleTime=-1  T=tsamp
  Out : Outport  OutDataType=fixdt(1,16,0)  OutScaling=[]
  wires:
  Actuator Trim/1 -> PID Controller/6(IniCond)
  Limits/1 -> PID Controller/5(Limits)
  Gains/1 -> PID Controller/4(Gains)
  State/1 -> PID Controller/3(State)
  PID Controller/1(Output) -> Out/1
  Rate Limit Ex/1 -> PID Controller/2(Cmd)
  Input/1 -> PID Controller/1(Input)
  50 [Pa/s]/1 -> Rate Limit Ex/2
  Cmd/1 -> Rate Limit Ex/1

== system PositionComplementary/Subsystem3/Autopilot/Pitch Control  Vector Inputs/Pitch Angle Hold ==
  note: Controller which takes in pitch rate and pitch angle and outputs elevator. The integral term is not used. Yet.
  Pitch angle : Inport
  Pitch rate : Inport  Port=2
  Pitch angle cmd : Inport  Port=3
  Pitch rate cmd : Inport  Port=4
  State : Inport  Port=5
  Gains : Inport  Port=6
  Demux1 : Demux  Outputs=3
  Demux5 : Demux  Outputs=3
  Derivative Gain : Product  Inputs=3  SaturateOnIntegerOverflow=on  InputSameDT=on
  Low-pass Filter : piccolo_library/Filters/Low-pass Filter  SystemSampleTime=-1  f=3  t=tsamp
  Proportional Gain : Product  Inputs=3  SaturateOnIntegerOverflow=on  InputSameDT=on
  Scope : Scope  NumInputPorts=5
      settings: YMin=-1~-0.075~-0.075~-5e+006~-5e+006  YMax=1~0.1~0.1~3.5e+007~3.5e+007  SaveName=ScopeData5
  Sum : Sum  SaturateOnIntegerOverflow=on  InputSameDT=on
  Sum1 : Sum  Inputs=|+-  SaturateOnIntegerOverflow=on  InputSameDT=on
  Sum2 : Sum  Inputs=|+-  SaturateOnIntegerOverflow=on  InputSameDT=on
  Terminator : Terminator
  Terminator1 : Terminator
  Out : Outport  OutDataType=fixdt(1,16,0)  OutScaling=[]
  wires:
  Demux1/2 -> Terminator1/1
  Demux1/1 -> Proportional Gain/3
  Demux1/3 -> Derivative Gain/3
  State/1 -> Demux1/1
  Demux5/2 -> Terminator/1
  Sum/1 -> Out/1, Scope/4
  Derivative Gain/1 -> Sum/2
  Proportional Gain/1 -> Sum/1, Scope/5
  Demux5/3 -> Derivative Gain/2
  Low-pass Filter/1 -> Derivative Gain/1
  Demux5/1 -> Proportional Gain/2
  Sum2/1 -> Proportional Gain/1, Scope/3
  Sum1/1 -> Low-pass Filter/1
  Pitch angle cmd/1 -> Sum2/2, Scope/1
  Pitch angle/1 -> Sum2/1, Scope/2
  Gains/1 -> Demux5/1
  Pitch rate/1 -> Sum1/1
  Pitch rate cmd/1 -> Sum1/2

== system PositionComplementary/Subsystem3/Autopilot/Roll Control Vector Inputs/Bank Angle Hold ==
  note: Controller which takes in roll rate and roll angle and outputs aileron.  Note that the derivative
      | term is simply the roll rate rather than the derivative of the error signal.
      | This is for backward compatible systems which aren't using the attitude data.
  note: pid
  Roll Rate : Inport
  Roll Angle : Inport  Port=2
  Cmd : Inport  Port=3
  State : Inport  Port=4
  Gains : Inport  Port=5
  Limits : Inport  Port=6
  IniCond : Inport  Port=7
  Demux1 : Demux  Outputs=3
  Demux2 : Demux  Outputs=3
  Derivative Gain : Product  Inputs=3  SaturateOnIntegerOverflow=on  InputSameDT=on
  Extended Integrator : piccolo_library/Integrators/Extended Integrator  SystemSampleTime=-1  T=tsamp
  Low-pass Filter : piccolo_library/Filters/Low-pass Filter  SystemSampleTime=-1  f=3  t=tsamp
  Proportional Gain : Product  Inputs=3  SaturateOnIntegerOverflow=on  InputSameDT=on
  Scope : Scope  NumInputPorts=10
      settings: YMin=-1~-0.07~-0.07~-0.02~-1~-1~-1~-1~-1~-1  YMax=1~0.03~0.03~0.07~1~1~1~1~1~1
  Sum2 : Sum  Inputs=+++  SaturateOnIntegerOverflow=on  InputSameDT=on
  Sum3 : Sum  Inputs=|+-  SaturateOnIntegerOverflow=on  InputSameDT=on
  Out : Outport  OutDataType=fixdt(1,16,0)  OutScaling=[]
  wires:
  Demux2/3 -> Derivative Gain/3
  Demux2/2 -> Extended Integrator/3
  Demux2/1 -> Proportional Gain/3
  State/1 -> Demux2/1
  Roll Rate/1 -> Low-pass Filter/1
  Low-pass Filter/1 -> Derivative Gain/1
  Demux1/2 -> Extended Integrator/4
  Sum2/1 -> Out/1, Scope/4
  Derivative Gain/1 -> Sum2/3, Scope/6  "derv"
  Extended Integrator/1 -> Sum2/2, Scope/5  "int"
  Proportional Gain/1 -> Sum2/1
  Demux1/3 -> Derivative Gain/2
  Demux1/1 -> Proportional Gain/2
  Limits/1 -> Extended Integrator/5
  IniCond/1 -> Extended Integrator/2
  Sum3/1 -> Extended Integrator/1, Proportional Gain/1, Scope/3  "err"
  Gains/1 -> Demux1/1
  Roll Angle/1 -> Scope/2, Sum3/1  "roll"
  Cmd/1 -> Sum3/2, Scope/1  "cmd"

== system PositionComplementary/Subsystem3/Autopilot/Roll Control Vector Inputs/Damper switch ==
  note: Select whether the individual components of the pitch and roll damper  loops are enabled or disabled.
      | This is done based on the specific loop enable state, the global state, and the mode of the autopilot.
      |
      | Note the use of the multiport  switch.  This switch is one based, and will truncate floating point
      | numbers.  Hence we add by 1.1 to guarantee we don't get the wrong state based on rounding
      | error.
  Globals : Inport
  Loop : Inport  Port=2
  Climbout : Constant
  Convert to 1 based : Constant  Value=1.1
  Default : Constant
  Demux : Demux  Outputs=3
  Display1 : Display
  Display2 : Display
  Display3 : Display
  Final Approach : Constant
  Flying : Constant
  Global and Loop on/off : Product  SaturateOnIntegerOverflow=on
  Land pattern : Constant
  Loop on or off : Switch  Threshold=0.5  SaturateOnIntegerOverflow=on
  Mux : Mux  Inputs=3
  Mux1 : Mux  Inputs=3
  Pre launch : Constant  Value=0
  Proportional\ Integral switch : MultiPortSwitch  Inputs=8  SaturateOnIntegerOverflow=on  InputSameDT=on
  Sum : Sum  Inputs=++|  SaturateOnIntegerOverflow=on  InputSameDT=on
  Terminator : Terminator
  Touchdown : Constant
  Transition : Constant  Value=0
  Zero : Constant  Value=0
  TriOut : Outport  OutDataType=fixdt(1,16,0)  OutScaling=[]
  wires:
  Default/1 -> Proportional\ Integral switch/9
  Touchdown/1 -> Proportional\ Integral switch/8
  Demux/3 -> Terminator/1
  Mux1/1 -> Loop on or off/1
  Proportional\ Integral switch/1 -> Mux1/3, Mux1/2, Mux1/1
  Final Approach/1 -> Proportional\ Integral switch/7
  Land pattern/1 -> Proportional\ Integral switch/6
  Flying/1 -> Proportional\ Integral switch/5
  Transition/1 -> Proportional\ Integral switch/3
  Climbout/1 -> Proportional\ Integral switch/4
  Pre launch/1 -> Proportional\ Integral switch/2
  Convert to 1 based/1 -> Sum/1
  Demux/2 -> Sum/2
  Sum/1 -> Proportional\ Integral switch/1
  Global and Loop on/off/1 -> Loop on or off/2, Display2/1
  Loop/1 -> Global and Loop on/off/2, Display3/1
  Demux/1 -> Global and Loop on/off/1, Display1/1
  Globals/1 -> Demux/1
  Zero/1 -> Mux/3, Mux/2, Mux/1
  Mux/1 -> Loop on or off/3
  Loop on or off/1 -> TriOut/1

== system PositionComplementary/Subsystem3/Autopilot/Roll Control Vector Inputs/Turn Rate Hold ==
  note: Standard PID feedback controller with integrator saturation. There are three gains, and three states, one for each term
  Input : Inport
  Cmd : Inport  Port=2
  State : Inport  Port=3
  Gains : Inport  Port=4
  Limits : Inport  Port=5
  IniCond : Inport  Port=6
  Demux : Demux  Outputs=3
  Demux1 : Demux  Outputs=3
  Derivative Gain : Product  Inputs=3  SaturateOnIntegerOverflow=on  InputSameDT=on
  Extended Integrator : piccolo_library/Integrators/Extended Integrator  SystemSampleTime=-1  T=tsamp
  Proportional Gain : Product  Inputs=3  SaturateOnIntegerOverflow=on  InputSameDT=on
  Scope1 : Scope  NumInputPorts=5
      settings: YMin=0.09325~0.09~-0.005~-1~-1  YMax=0.09475~0.1075~0.0125~1~1  SaveName=ScopeData25
  Sum : Sum  Inputs=|+-  SaturateOnIntegerOverflow=on
  Sum3 : Sum  Inputs=+++  SaturateOnIntegerOverflow=on  InputSameDT=on
  dx/dt with TD : piccolo_library/Derivatives/dx//dt with TD  SystemSampleTime=-1  tsamp=tsamp  tdelay=tdelay
  Output : Outport  OutDataType=fixdt(1,16,0)  OutScaling=[]
  wires:
  Sum3/1 -> Output/1, Scope1/4
  Demux1/3 -> Derivative Gain/3
  Demux1/2 -> Extended Integrator/3
  Demux1/1 -> Proportional Gain/3
  State/1 -> Demux1/1
  IniCond/1 -> Extended Integrator/2
  Limits/1 -> Extended Integrator/5
  Demux/2 -> Extended Integrator/4
  Extended Integrator/1 -> Sum3/2
  Derivative Gain/1 -> Sum3/3
  Proportional Gain/1 -> Sum3/1
  Demux/3 -> Derivative Gain/2
  Demux/1 -> Proportional Gain/2
  Gains/1 -> Demux/1
  dx/dt with TD/1 -> Derivative Gain/1
  Sum/1 -> Extended Integrator/1, dx/dt with TD/1, Scope1/3, Proportional Gain/1
  Cmd/1 -> Sum/2, Scope1/1
  Input/1 -> Sum/1, Scope1/2

== system PositionComplementary/Subsystem3/L1 Adaptive Controller LATERAL-DIRECTIONAL/PF Yaw Channel L1 Augmentation/Adaptive Law ==
  u_psi_tilda : Inport
  Integrator : Integrator  LimitOutput=on  UpperSaturationLimit=Pbound  LowerSaturationLimit=-Pbound
  ON : Constant  Value=gamma
  Projection : Product  RndMeth=Zero
  Scope1 : Scope  NumInputPorts=3
      settings: YMin=-0.1~-0.004~-6  YMax=0.1~0.003~8  SaveName=ScopeData27
  sighat_2 : Outport
  wires:
  Integrator/1 -> sighat_2/1, Scope1/1
  ON/1 -> Projection/1
  Projection/1 -> Integrator/1, Scope1/3
  u_psi_tilda/1 -> Projection/2, Scope1/2  "u_psi_tilda"

== system PositionComplementary/Subsystem3/L1 Adaptive Controller LATERAL-DIRECTIONAL/PF Yaw Channel L1 Augmentation/C(s) ==
  sighat_2 : Inport
  Integrator2 : Integrator
  ON : Constant  Value=omega
  Product : Product  RndMeth=Zero
  Sum2 : Sum  Inputs=|+-
  C_sighat_2 : Outport
  wires:
  Integrator2/1 -> C_sighat_2/1, Sum2/2
  Sum2/1 -> Product/2
  Product/1 -> Integrator2/1
  sighat_2/1 -> Sum2/1
  ON/1 -> Product/1

== system PositionComplementary/Subsystem3/L1 Adaptive Controller LATERAL-DIRECTIONAL/PF Yaw Channel L1 Augmentation/State predictor ==
  u2 : Inport
  sighat_2 : Inport  Port=2
  Integrator2 : Integrator
  ON : Constant  Value=m
  Product : Product  RndMeth=Zero
  Sum1 : Sum  Inputs=|++
  Sum2 : Sum  Inputs=|+-
  u_psi_hat : Outport
  wires:
  sighat_2/1 -> Sum1/2
  Sum1/1 -> Sum2/1
  u2/1 -> Sum1/1
  Integrator2/1 -> u_psi_hat/1, Sum2/2
  Sum2/1 -> Product/2
  Product/1 -> Integrator2/1
  ON/1 -> Product/1

== system PositionComplementary/Subsystem3/L1 Adaptive Controller LONGITUDINAL/PF Yaw Channel L1 Augmentation/Adaptive Law ==
  u_psi_tilda : Inport
  Integrator : Integrator  LimitOutput=on  UpperSaturationLimit=Pbound  LowerSaturationLimit=-Pbound
  ON : Constant  Value=gamma
  Projection : Product  RndMeth=Zero
  Scope1 : Scope  NumInputPorts=3
      settings: TimeRange=4  YMin=-0.1~-1000~-6  YMax=0.1~200~8  SaveName=ScopeData27
  sighat_2 : Outport
  wires:
  u_psi_tilda/1 -> Scope1/2, Projection/2  "u_psi_tilda"
  Projection/1 -> Scope1/3, Integrator/1
  ON/1 -> Projection/1
  Integrator/1 -> Scope1/1, sighat_2/1

== system PositionComplementary/Subsystem3/L1 Adaptive Controller LONGITUDINAL/PF Yaw Channel L1 Augmentation/C(s) ==
  sighat_2 : Inport
  Integrator2 : Integrator
  ON : Constant  Value=omega
  Product : Product  RndMeth=Zero
  Sum2 : Sum  Inputs=|+-
  C_sighat_2 : Outport
  wires:
  ON/1 -> Product/1
  sighat_2/1 -> Sum2/1
  Product/1 -> Integrator2/1
  Sum2/1 -> Product/2
  Integrator2/1 -> Sum2/2, C_sighat_2/1

== system PositionComplementary/Subsystem3/L1 Adaptive Controller LONGITUDINAL/PF Yaw Channel L1 Augmentation/State predictor ==
  u2 : Inport
  sighat_2 : Inport  Port=2
  Integrator2 : Integrator
  ON : Constant  Value=m
  Product : Product  RndMeth=Zero
  Sum1 : Sum  Inputs=|++
  Sum2 : Sum  Inputs=|+-
  u_psi_hat : Outport
  wires:
  ON/1 -> Product/1
  Product/1 -> Integrator2/1
  Sum2/1 -> Product/2
  Integrator2/1 -> Sum2/2, u_psi_hat/1
  u2/1 -> Sum1/1
  Sum1/1 -> Sum2/1
  sighat_2/1 -> Sum1/2

== system PositionComplementary/Attitude Complementary Filter/Subsystem/get Centripetal/3vector LPF/Low Pass1 ==
  In1 : Inport
  Discrete Zero-Pole : DiscreteZeroPole  Zeros=zerosd  Poles=polesd  Gain=gaind  SampleTime=SampleTime
  Out1 : Outport
  wires:
  In1/1 -> Discrete Zero-Pole/1
  Discrete Zero-Pole/1 -> Out1/1

== system PositionComplementary/Attitude Complementary Filter/Subsystem/get Centripetal/3vector LPF/Low Pass2 ==
  In1 : Inport
  Discrete Zero-Pole : DiscreteZeroPole  Zeros=zerosd  Poles=polesd  Gain=gaind  SampleTime=SampleTime
  Out1 : Outport
  wires:
  Discrete Zero-Pole/1 -> Out1/1
  In1/1 -> Discrete Zero-Pole/1

== system PositionComplementary/Attitude Complementary Filter/Subsystem/get Centripetal/3vector LPF/Low Pass3 ==
  In1 : Inport
  Discrete Zero-Pole : DiscreteZeroPole  Zeros=zerosd  Poles=polesd  Gain=gaind  SampleTime=SampleTime
  Out1 : Outport
  wires:
  In1/1 -> Discrete Zero-Pole/1
  Discrete Zero-Pole/1 -> Out1/1
